simulink model "HIL_Testing_SW"  (Simulink 7.5)
settings: Solver=ode1  StartTime=0.0  StopTime=Inf  FixedStep=0.001  RelTol=1e-3
PostLoadFcn:
  | , if any(exist('dsrtsu_mdlpostloadfcn', 'file') == [2, 3, 6]), try dsrtsu_mdlpostloadfcn('Execute', bdroot); catch fprintf('Error in PostLoadFcn (dsrtsu_mdlpostloadfcn) for model "%s":\n %s\n', bdroot, lasterr); end, end,
undefined symbols (not defined in the file): CeBSER_Cnt_NumTempAxisPts, ChargeCord, ChargeCord_Control, ChargeToSOCCurr, ChrgCurrLim, CrntSens1Fine, CS_SOCSetPt, CyclerMaxChrgPwr, CyclerMaxDschrgPwr, deltaAhr, Drive_1, Drive_10, Drive_11, Drive_12, Drive_13, Drive_14, Drive_15, Drive_16, Drive_17, Drive_18, Drive_19, Drive_2, Drive_20, Drive_21, Drive_22, Drive_23, Drive_24, Drive_25, Drive_26, Drive_27, Drive_28, Drive_29, Drive_3, Drive_30, Drive_31, Drive_32, Drive_33, Drive_34, Drive_35, Drive_36, Drive_37, Drive_38, Drive_39, Drive_4, Drive_40, Drive_41, Drive_42, Drive_43, Drive_44, Drive_45, Drive_46, Drive_47, Drive_48, Drive_49, Drive_5, Drive_50, Drive_51, Drive_6, Drive_7, Drive_8 ... (+50)
libraries: simulink x129, rtican x50, rti2211sailib x5, rti2211serlib x5, rti2202miolib x3
(part 3 of 23)

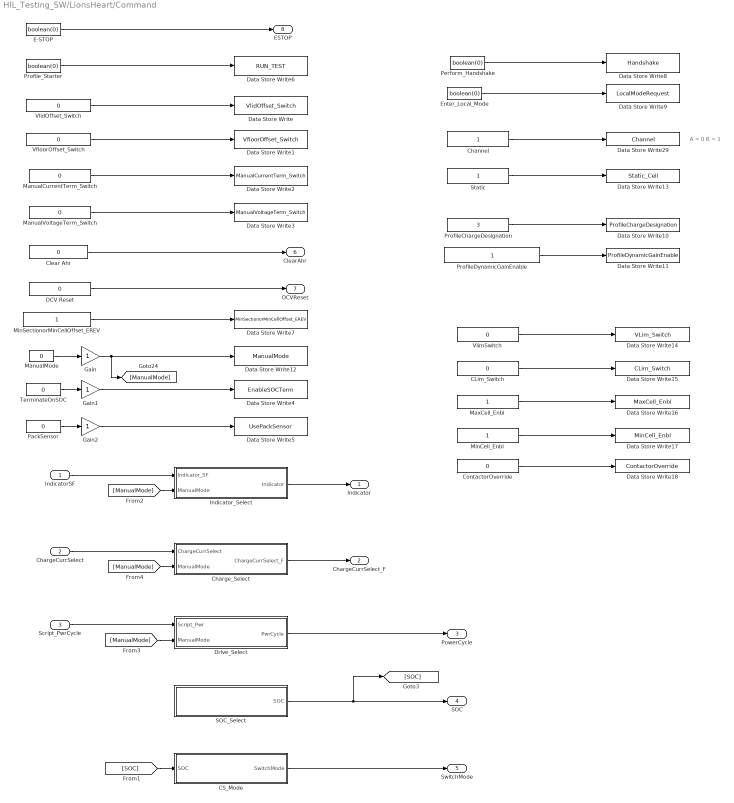
== system HIL_Testing_SW/LionsHeart/Command ==
  note: A = 0
      | B = 1
  IndicatorSF : Inport  OutDataType=fixdt(1, 16)  OutScaling=2^0
  ChargeCurrSelect : Inport  Port=2  OutDataType=fixdt(1, 16)  OutScaling=2^0
  Script_PwrCycle : Inport  Port=3  OutDataType=fixdt(1, 16)  OutScaling=2^0
  CLim_Switch : Constant  Value=0  OutDataType=sfix(16)  OutScaling=2^0
  CS_Mode : Subsystem
  Channel : Constant  OutDataTypeMode=double  OutDataType=sfix(16)  OutScaling=2^0  OutDataTypeStr=double
  Charge_Select : Subsystem
  Clear Ahr : Constant  Value=0  OutDataTypeMode=boolean  OutDataType=fixdt(1, 16)  OutScaling=2^0  OutDataTypeStr=boolean
  ContactorOverride : Constant  Value=0  OutDataType=sfix(16)  OutScaling=2^0
  Data Store Write : DataStoreWrite  DataStoreName=VlidOffset_Switch  SampleTime=-1
  Data Store Write1 : DataStoreWrite  DataStoreName=VfloorOffset_Switch  SampleTime=-1
  Data Store Write10 : DataStoreWrite  DataStoreName=ProfileChargeDesignation  SampleTime=-1
  Data Store Write11 : DataStoreWrite  DataStoreName=ProfileDynamicGainEnable  SampleTime=-1
  Data Store Write12 : DataStoreWrite  DataStoreName=ManualMode  SampleTime=-1
  Data Store Write13 : DataStoreWrite  DataStoreName=Static_Cell  SampleTime=-1
  Data Store Write14 : DataStoreWrite  DataStoreName=VLim_Switch  SampleTime=-1
  Data Store Write15 : DataStoreWrite  DataStoreName=CLim_Switch  SampleTime=-1
  Data Store Write16 : DataStoreWrite  DataStoreName=MaxCell_Enbl  SampleTime=-1
  Data Store Write17 : DataStoreWrite  DataStoreName=MinCell_Enbl  SampleTime=-1
  Data Store Write18 : DataStoreWrite  DataStoreName=ContactorOverride  SampleTime=-1
  Data Store Write2 : DataStoreWrite  DataStoreName=ManualCurrentTerm_Switch  SampleTime=-1
  Data Store Write29 : DataStoreWrite  DataStoreName=Channel  SampleTime=-1
  Data Store Write3 : DataStoreWrite  DataStoreName=ManualVoltageTerm_Switch  SampleTime=-1
  Data Store Write4 : DataStoreWrite  DataStoreName=EnableSOCTerm  SampleTime=-1
  Data Store Write5 : DataStoreWrite  DataStoreName=UsePackSensor  SampleTime=-1
  Data Store Write6 : DataStoreWrite  DataStoreName=RUN_TEST  SampleTime=-1
  Data Store Write7 : DataStoreWrite  DataStoreName=MinSectionorMinCellOffset_EREV  SampleTime=-1
  Data Store Write8 : DataStoreWrite  DataStoreName=Handshake  SampleTime=-1
  Data Store Write9 : DataStoreWrite  DataStoreName=LocalModeRequest  SampleTime=-1
  Drive_Select : Subsystem
  E-STOP : Constant  Value=boolean(0)  OutDataType=sfix(16)  OutScaling=2^0
  Enter_Local_Mode : Constant  Value=boolean(0)  OutDataType=sfix(16)  OutScaling=2^0
  Gain : Gain  ParameterDataType=sfix(16)  ParameterScaling=2^0  OutDataType=sfix(16)  OutScaling=2^0
  Gain1 : Gain  ParameterDataType=sfix(16)  ParameterScaling=2^0  OutDataType=sfix(16)  OutScaling=2^0  OutDataTypeStr=Inherit: Same as input
  Gain2 : Gain  ParameterDataType=sfix(16)  ParameterScaling=2^0  OutDataType=sfix(16)  OutScaling=2^0  OutDataTypeStr=Inherit: Same as input
  Indicator_Select : Subsystem
  ManualCurrentTerm_Switch : Constant  Value=0  OutDataTypeMode=double  OutDataType=sfix(16)  OutScaling=2^0  OutDataTypeStr=double
  ManualMode : Constant  Value=0  OutDataType=fixdt(1, 16)  OutScaling=2^0
  ManualVoltageTerm_Switch : Constant  Value=0  OutDataType=sfix(16)  OutScaling=2^0
  MaxCell_Enbl : Constant  OutDataType=sfix(16)  OutScaling=2^0
  MinCell_Enbl : Constant  OutDataType=sfix(16)  OutScaling=2^0
  MinSectionorMinCellOffset_EREV : Constant  OutDataType=fixdt(1, 16)  OutScaling=2^0
  OCV Reset : Constant  Value=0  OutDataTypeMode=boolean  OutDataType=fixdt(1, 16)  OutScaling=2^0  OutDataTypeStr=boolean
  PackSensor : Constant  Value=0  OutDataTypeMode=boolean  OutDataType=sfix(16)  OutScaling=2^0  OutDataTypeStr=boolean
  Perform_Handshake : Constant  Value=boolean(0)  OutDataType=sfix(16)  OutScaling=2^0
  ProfileChargeDesignation : Constant  Value=3  OutDataType=sfix(16)  OutScaling=2^0
  ProfileDynamicGainEnable : Constant  OutDataType=sfix(16)  OutScaling=2^0
  Profile_Starter : Constant  Value=boolean(0)  OutDataType=sfix(16)  OutScaling=2^0
  SOC_Select : Subsystem
  Static : Constant  OutDataTypeMode=double  OutDataType=sfix(16)  OutScaling=2^0  OutDataTypeStr=double
  TerminateOnSOC : Constant  Value=0  OutDataTypeMode=boolean  OutDataType=sfix(16)  OutScaling=2^0  OutDataTypeStr=boolean
  VfloorOffset_Switch : Constant  Value=0  OutDataType=fixdt(1, 16)  OutScaling=2^0
  VlidOffset_Switch : Constant  Value=0  OutDataType=fixdt(1, 16)  OutScaling=2^0
  VlimSwitch : Constant  Value=0  OutDataType=sfix(16)  OutScaling=2^0
  Indicator : Outport  OutDataType=fixdt(1, 16)  OutScaling=2^0
  ChargeCurrSelect_F : Outport  Port=2  OutDataType=fixdt(1, 16)  OutScaling=2^0
  PowerCycle : Outport  Port=3  OutDataType=fixdt(1, 16)  OutScaling=2^0
  SOC : Outport  Port=4  OutDataType=fixdt(1, 16)  OutScaling=2^0
  SwitchMode : Outport  Port=5  OutDataType=fixdt(1, 16)  OutScaling=2^0
  ClearAhr : Outport  Port=6  OutDataType=fixdt(1, 16)  OutScaling=2^0
  OCVReset : Outport  Port=7  OutDataType=fixdt(1, 16)  OutScaling=2^0
  ESTOP : Outport  Port=8  OutDataType=fixdt(1, 16)  OutScaling=2^0
  wires:
  E-STOP/1 -> ESTOP/1
  Profile_Starter/1 -> Data Store Write6/1
  ManualMode/1 -> Gain/1
  SOC_Select/1(SOC) -> SOC/1, [SOC]
  PackSensor/1 -> Gain2/1
  TerminateOnSOC/1 -> Gain1/1
  [SOC] -> CS_Mode/1(SOC)
  CS_Mode/1(SwitchMode) -> SwitchMode/1
  Gain/1 -> [ManualMode], Data Store Write12/1
  Script_PwrCycle/1 -> Drive_Select/1(Script_Pwr)
  Drive_Select/1(PwrCycle) -> PowerCycle/1
  [ManualMode] -> Drive_Select/2(ManualMode)
  ChargeCurrSelect/1 -> Charge_Select/1(ChargeCurrSelect)
  [ManualMode] -> Charge_Select/2(ManualMode)
  Charge_Select/1(ChargeCurrSelect_F) -> ChargeCurrSelect_F/1
  IndicatorSF/1 -> Indicator_Select/1(Indicator_SF)
  Indicator_Select/1(Indicator) -> Indicator/1
  [ManualMode] -> Indicator_Select/2(ManualMode)
  VlidOffset_Switch/1 -> Data Store Write/1
  VfloorOffset_Switch/1 -> Data Store Write1/1
  ManualCurrentTerm_Switch/1 -> Data Store Write2/1
  ManualVoltageTerm_Switch/1 -> Data Store Write3/1
  Gain1/1 -> Data Store Write4/1
  Gain2/1 -> Data Store Write5/1
  Clear Ahr/1 -> ClearAhr/1
  OCV Reset/1 -> OCVReset/1
  MinSectionorMinCellOffset_EREV/1 -> Data Store Write7/1
  Perform_Handshake/1 -> Data Store Write8/1
  Enter_Local_Mode/1 -> Data Store Write9/1
  Channel/1 -> Data Store Write29/1
  ProfileChargeDesignation/1 -> Data Store Write10/1
  ProfileDynamicGainEnable/1 -> Data Store Write11/1
  VlimSwitch/1 -> Data Store Write14/1
  CLim_Switch/1 -> Data Store Write15/1
  MaxCell_Enbl/1 -> Data Store Write16/1
  MinCell_Enbl/1 -> Data Store Write17/1
  ContactorOverride/1 -> Data Store Write18/1
  Static/1 -> Data Store Write13/1

== system HIL_Testing_SW/LionsHeart/FeaturePresentation ==
  CyclerVoltage : Inport  OutDataType=fixdt(1, 16)  OutScaling=2^0
  BatTemp : Inport  Port=2  OutDataType=fixdt(1, 16)  OutScaling=2^0
  ClearAhr : Inport  Port=3  OutDataType=fixdt(1, 16)  OutScaling=2^0
  PackCurrent : Inport  Port=4  OutDataType=fixdt(1, 16)  OutScaling=2^0
  CyclerCurrent : Inport  Port=5  OutDataType=fixdt(1, 16)  OutScaling=2^0
  PackVoltage : Inport  Port=6  OutDataType=fixdt(1, 16)  OutScaling=2^0
  OCVReset : Inport  Port=7  OutDataType=fixdt(1, 16)  OutScaling=2^0
  PackVolt_MinCell : Inport  Port=8  OutDataType=fixdt(1, 16)  OutScaling=2^0
  PackVolt_MaxCell : Inport  Port=9  OutDataType=fixdt(1, 16)  OutScaling=2^0
  Indicator : Inport  Port=10  OutDataType=fixdt(1, 16)  OutScaling=2^0
  CS_SwitchMode : Inport  Port=11  OutDataType=fixdt(1, 16)  OutScaling=2^0
  ESTOP : Inport  Port=12  OutDataType=fixdt(1, 16)  OutScaling=2^0
  ChrgCurrSelect_F : Inport  Port=13  OutDataType=fixdt(1, 16)  OutScaling=2^0
  SOC : Inport  Port=14  OutDataType=fixdt(1, 16)  OutScaling=2^0
  PwrCycle : Inport  Port=15  OutDataType=fixdt(1, 16)  OutScaling=2^0
  ContactorStatus : Inport  Port=16  OutDataType=fixdt(1, 16)  OutScaling=2^0
  Voltage_Cntrl : Inport  Port=17  OutDataType=fixdt(1, 16)  OutScaling=2^0
  Current_Cntrl : Inport  Port=18  OutDataType=fixdt(1, 16)  OutScaling=2^0
  Ahr_Integration : Subsystem
  Down_to_Business : Subsystem
  Safety : Subsystem
  Profile_Control_Value : Outport  OutDataType=fixdt(1, 16)  OutScaling=2^0
  ChargeMode : Outport  Port=2  OutDataType=fixdt(1, 16)  OutScaling=2^0
  Profile_Control_Mode : Outport  Port=3  OutDataType=fixdt(1, 16)  OutScaling=2^0
  VoltTarget : Outport  Port=4  OutDataType=fixdt(1, 16)  OutScaling=2^0
  IndicatorSF : Outport  Port=5  OutDataType=fixdt(1, 16)  OutScaling=2^0
  Script_PwrCycle : Outport  Port=6  OutDataType=fixdt(1, 16)  OutScaling=2^0
  ChargeCurrSelect : Outport  Port=7  OutDataType=fixdt(1, 16)  OutScaling=2^0
  SetChamberT_ToBatTemp : Outport  Port=8  OutDataType=fixdt(1, 16)  OutScaling=2^0
  wires:
  Safety/1(Control_Mode_Proc) -> Profile_Control_Mode/1
  Down_to_Business/1(Profile_Data) -> Profile_Control_Value/1
  Down_to_Business/2(CM) -> ChargeMode/1, [ChargeMode]
  Down_to_Business/3(ResetSOC) -> [ResetSOC]
  Down_to_Business/4(VoltTarget) -> VoltTarget/1
  Down_to_Business/5(IndicatorSF) -> IndicatorSF/1
  Down_to_Business/6(Profile_Mode) -> [Profile_Mode]
  [BatTemp] -> Safety/1(BatTemp)
  [PackVolt_MinCell] -> Safety/2(PackVolt_MinCell)
  [PackVolt_MaxCell] -> Safety/3(PackVolt_MaxCell)
  [Profile_Mode] -> Safety/4(Mode)
  [ChargeMode] -> Safety/6(ChargeMode)
  [CyclerVoltage] -> Safety/8(CyclerVoltage)
  [Indicator] -> Safety/7(Indicator)
  OCVReset/1 -> Ahr_Integration/8(OCVReset)
  ClearAhr/1 -> Ahr_Integration/3(ClearAhr)
  [ResetSOC] -> Ahr_Integration/4(ResetSOC)
  CyclerVoltage/1 -> [CyclerVoltage]
  BatTemp/1 -> [BatTemp]
  PackCurrent/1 -> [PackCurrent]
  CyclerCurrent/1 -> [CyclerCurrent]
  PackVoltage/1 -> [PackVoltage]
  [CyclerVoltage] -> Ahr_Integration/1(CyclerVoltage)
  [BatTemp] -> Ahr_Integration/2(BatTemp)
  [PackCurrent] -> Ahr_Integration/5(PackCurrent)
  [CyclerCurrent] -> Ahr_Integration/6(CyclerCurrent)
  [PackVoltage] -> Ahr_Integration/7(PackVoltage)
  [CyclerCurrent] -> Down_to_Business/1(CyclerCurrent)
  [CyclerVoltage] -> Down_to_Business/2(CyclerVoltage)
  [BatTemp] -> Down_to_Business/3(BatTemp)
  [PackVoltage] -> Down_to_Business/4(PackVoltage)
  [PackCurrent] -> Down_to_Business/5(PackCurrent)
  PackVolt_MinCell/1 -> [PackVolt_MinCell]
  PackVolt_MaxCell/1 -> [PackVolt_MaxCell]
  [PackVolt_MaxCell] -> Down_to_Business/6(PackVolt_MaxCell)
  [PackVolt_MinCell] -> Down_to_Business/7(PackVolt_MinCell)
  Indicator/1 -> Down_to_Business/8(Indicator), [Indicator]
  CS_SwitchMode/1 -> Down_to_Business/9(CS_SwitchMode)
  ESTOP/1 -> Down_to_Business/10(ESTOP)
  ContactorStatus/1 -> Safety/5(ContactorStatus)
  ChrgCurrSelect_F/1 -> Down_to_Business/11(ChrgCurrSelect_F)
  SOC/1 -> Down_to_Business/12(SOC)
  PwrCycle/1 -> Down_to_Business/13(PwrCycle)
  Down_to_Business/7(Script_PwrCycle) -> Script_PwrCycle/1
  Down_to_Business/8(ChargeCurrSelect) -> ChargeCurrSelect/1
  [PackVoltage] -> Safety/9(PackVoltage)
  Voltage_Cntrl/1 -> Down_to_Business/14(Voltage_Cntrl)
  Current_Cntrl/1 -> Down_to_Business/15(Current_Cntrl)
  Down_to_Business/9(SetChamberT_ToBatTemp) -> SetChamberT_ToBatTemp/1

== system HIL_Testing_SW/LionsHeart/Input Processing ==
  MinCell : Inport  OutDataType=fixdt(1, 16)  OutScaling=2^0
  MaxCell : Inport  Port=2  OutDataType=fixdt(1, 16)  OutScaling=2^0
  BatTemp : Inport  Port=3  OutDataType=fixdt(1, 16)  OutScaling=2^0
  MinSectionVoltage : Inport  Port=4  OutDataType=fixdt(1, 16)  OutScaling=2^0
  VoltTarget : Inport  Port=5  OutDataType=fixdt(1, 16)  OutScaling=2^0
  PackVoltage : Inport  Port=6  OutDataType=fixdt(1, 16)  OutScaling=2^0
  Timestamp : Inport  Port=7  OutDataType=fixdt(1, 16)  OutScaling=2^0
  CyclerCurrent : Inport  Port=8  OutDataType=fixdt(1, 16)  OutScaling=2^0
  CyclerVotlage : Inport  Port=9  OutDataType=fixdt(1, 16)  OutScaling=2^0
  HVBatVltLwLmt_CAN : Inport  Port=10  OutDataType=fixdt(1, 16)  OutScaling=2^0
  HVBatVltUpLmt_CAN : Inport  Port=11  OutDataType=fixdt(1, 16)  OutScaling=2^0
  HVBatCrntLwLmt_CAN : Inport  Port=12  OutDataType=fixdt(1, 16)  OutScaling=2^0
  HVBatCrntUpLmt_CAN : Inport  Port=13  OutDataType=fixdt(1, 16)  OutScaling=2^0
  PackCurrent : Inport  Port=14  OutDataType=fixdt(1, 16)  OutScaling=2^0
  Current Processing : Subsystem
  Power : Subsystem
  Time : Subsystem
  Voltage Processing : Subsystem
  PackVolt_MinCell : Outport  OutDataType=fixdt(1, 16)  OutScaling=2^0
  PackVolt_MaxCell : Outport  Port=2  OutDataType=fixdt(1, 16)  OutScaling=2^0
  Voltage_Cntrl : Outport  Port=3  OutDataType=fixdt(1, 16)  OutScaling=2^0
  Current_Cntrl : Outport  Port=4  OutDataType=fixdt(1, 16)  OutScaling=2^0
  wires:
  Voltage Processing/1(PackVolt_MinCell) -> PackVolt_MinCell/1
  Voltage Processing/2(PackVolt_MaxCell) -> PackVolt_MaxCell/1
  MinCell/1 -> Voltage Processing/1(MinCell)
  MaxCell/1 -> Voltage Processing/2(MaxCell)
  MinSectionVoltage/1 -> Voltage Processing/4(MinSectionVoltage_EREV)
  VoltTarget/1 -> Voltage Processing/5(VoltageTarget)
  BatTemp/1 -> [BatTemp]
  [BatTemp] -> Voltage Processing/3(BatteryTemp)
  [BatTemp] -> Current Processing/1(BatteryTemp)
  Timestamp/1 -> Time/1(Timestamp_A)
  PackVoltage/1 -> Voltage Processing/6(PackVoltage)
  HVBatVltLwLmt_CAN/1 -> Voltage Processing/7(HVBatVltLwLmt_CAN)
  HVBatVltUpLmt_CAN/1 -> Voltage Processing/8(HVBatVltUpLmt_CAN)
  HVBatCrntLwLmt_CAN/1 -> Current Processing/2(HVBatCrntLwLmt_CAN)
  HVBatCrntUpLmt_CAN/1 -> Current Processing/3(HVBatCrntUpLmt_CAN)
  CyclerCurrent/1 -> [CyclerCurrent]
  CyclerVotlage/1 -> [CyclerVoltage]
  [CyclerCurrent] -> Power/1(CyclerCurrent)
  [CyclerVoltage] -> Power/2(CyclerVoltage)
  Voltage Processing/3(Voltage_Cntrl) -> Voltage_Cntrl/1
  PackCurrent/1 -> Current Processing/4(PackCurrent)
  [CyclerCurrent] -> Current Processing/5(CyclerCurrent)
  [CyclerVoltage] -> Voltage Processing/9(CyclerVoltage)
  Current Processing/1(Current_Cntrl) -> Current_Cntrl/1

== system HIL_Testing_SW/LionsHeart/OutputProcessing ==
  note: 5 = PowerPulse, defaults to limiting power by BCPR Limits
  note: **Add ability to limit by ST and Inst powerlimits 11/14/2012
  Indicator : Inport  OutDataType=sfix(16)  OutScaling=2^0
  ControlValue : Inport  Port=2  OutDataType=sfix(16)  OutScaling=2^0
  ControlMode : Inport  Port=3  OutDataType=sfix(16)  OutScaling=2^0
  LT_PwrDschlmt : Inport  Port=4  OutDataType=sfix(16)  OutScaling=2^0
  LT_PwrChgLmt : Inport  Port=5  OutDataType=sfix(16)  OutScaling=2^0
  Apply_BSE_PowerLimits : Subsystem
  Compare To Constant5 : simulink/Logic and Bit Operations/Compare To Constant  SystemSampleTime=-1  relop===  const=5  LogicOutDataTypeMode=boolean
  Logical Operator : Logic  Operator=OR  AllPortsSameDT=off  OutDataTypeMode=boolean  OutDataTypeStr=boolean
  ManualPowerLimitsSwitch : Constant  Value=0  OutDataType=sfix(16)  OutScaling=2^0
  Control_Value_Proc : Outport  OutDataType=fixdt(1, 16)  OutScaling=2^0
  wires:
  Indicator/1 -> Compare To Constant5/1
  Compare To Constant5/1 -> Logical Operator/1
  ManualPowerLimitsSwitch/1 -> Logical Operator/2
  Logical Operator/1 -> Apply_BSE_PowerLimits/3(SwitchPowerLimit)
  Apply_BSE_PowerLimits/1(Control_Value_Proc) -> Control_Value_Proc/1
  ControlValue/1 -> Apply_BSE_PowerLimits/1(ControlValue)
  ControlMode/1 -> Apply_BSE_PowerLimits/5(ControlMode)
  LT_PwrDschlmt/1 -> Apply_BSE_PowerLimits/2(LT_PwrDschLmt)
  LT_PwrChgLmt/1 -> Apply_BSE_PowerLimits/4(LT_PwrChgLmt)

== system HIL_Testing_SW/RTI Data/RTI Data Store ==
  RTI Data Store : Subsystem
      mask Type: RTI_DATA_STORE
      mask Description:
      | RTI Data Store Block. This block is used by RTI to store internal model dependent data. Deleting this block will result in data loss.
      | 
      | NEVER DELETE, COPY, OR MODIFY THIS BLOCK!
      mask Help:
      | RTI Data Store Block. This block is used by RTI to store internal model dependent data. Deleting this block will result in data loss.
      | 
      | NEVER DELETE, COPY, OR MODIFY THIS BLOCK!
      mask Display: text(0.5, 0.5, ' ', 'HorizontalAlignment', 'center');

== system HIL_Testing_SW/RX/Read BAS3 ==
  Enable : EnablePort
  Data Store Read : DataStoreRead  DataStoreName=RUN  SampleTime=0
  Data Store Read1 : DataStoreRead  DataStoreName=ACC  SampleTime=0
  Logical Operator : Logic  Operator=OR  AllPortsSameDT=off  LogicDataType=fixdt(0, 8)
  PID_Reads : Subsystem
  Read PTEX : Subsystem
  LT_PwrDschLmt : Outport  OutDataType=sfix(16)  OutScaling=2^0
  LT_PwrChgLmt : Outport  Port=2  OutDataType=sfix(16)  OutScaling=2^0
  SOC : Outport  Port=3  OutDataType=sfix(16)  OutScaling=2^0
  MinCell : Outport  Port=4  OutDataType=sfix(16)  OutScaling=2^0
  MaxCell : Outport  Port=5  OutDataType=sfix(16)  OutScaling=2^0
  CntctrStat : Outport  Port=6  OutDataType=sfix(16)  OutScaling=2^0
  PackCurrent : Outport  Port=7  OutDataType=sfix(16)  OutScaling=2^0
  PackVoltage : Outport  Port=8  OutDataType=sfix(16)  OutScaling=2^0
  BatTemp : Outport  Port=9  OutDataType=sfix(16)  OutScaling=2^0
  HVBatVltUpLmt_CAN : Outport  Port=10  OutDataType=sfix(16)  OutScaling=2^0
  HVBatVltLwLmt_CAN : Outport  Port=11  OutDataType=sfix(16)  OutScaling=2^0
  HVBatCrmtLwLmt_CAN : Outport  Port=12  OutDataType=sfix(16)  OutScaling=2^0
  HVBatCrmtUpLmt_CAN : Outport  Port=13  OutDataType=sfix(16)  OutScaling=2^0
  wires:
  Read PTEX/1(LT_PwrDschLmt) -> LT_PwrDschLmt/1
  Read PTEX/2(LT_PwrChgLmt) -> LT_PwrChgLmt/1
  Read PTEX/3(SOC) -> SOC/1
  Read PTEX/4(Voltage) -> PackVoltage/1
  PID_Reads/1(MinCell) -> MinCell/1
  PID_Reads/2(MaxCell) -> MaxCell/1
  PID_Reads/3(BatTemp) -> BatTemp/1
  Read PTEX/5(PackCurrent) -> PackCurrent/1
  Read PTEX/6(ContactorStatus) -> CntctrStat/1
  Logical Operator/1 -> PID_Reads/Enable
  Data Store Read/1 -> Logical Operator/1
  Data Store Read1/1 -> Logical Operator/2
  Read PTEX/7(HVBatVltUpLmt_CAN) -> HVBatVltUpLmt_CAN/1
  Read PTEX/8(HVBatVltLwLmt_CAN) -> HVBatVltLwLmt_CAN/1
  Read PTEX/9(HVBatCrntLwLmt_CAN) -> HVBatCrmtLwLmt_CAN/1
  Read PTEX/10(HVBatCrntUpLmt_CAN) -> HVBatCrmtUpLmt_CAN/1
